simulink subsystem "EncondersHFz"  (R2023b)
settings: Solver=VariableStepAuto  StartTime=0.0  StopTime=10.0  RelTol=1e-3
libraries: arduinosensorlib x2, simulink x1
settings Model: Creator=Hajar  LastModifiedBy=Hajar

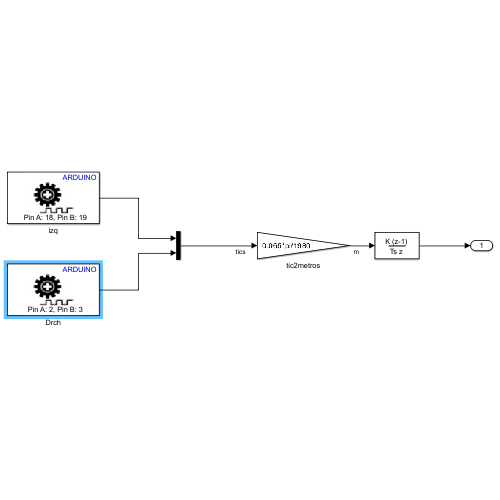
[thumbnail: Simulink's stored preview of the top-level diagram]
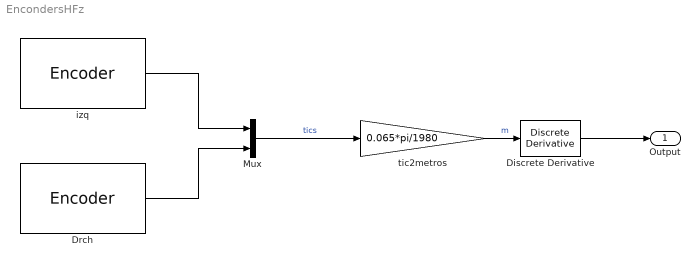
== system EncondersHFz ==
  Discrete Derivative : simulink/Discrete/Discrete Derivative  gainval=1.0  ICPrevScaledInput=0.0  OutMin=[]  OutMax=[]  OutDataType=fixdt(1, 16)  OutScaling=2^-10  DoSatur=off
  Drch : arduinosensorlib/Encoder  InputA=2  InputB=3  Mode=No reset  SampleTime=-1
  Mux : Mux  Inputs=2
  izq : arduinosensorlib/Encoder  InputA=18  InputB=19  Mode=No reset  SampleTime=-1
  tic2metros : Gain  Gain=0.065*pi/1980  OutDataTypeStr=double
  Output : Outport
  wires:
  izq/1 -> Mux/1
  Drch/1 -> Mux/2
  Mux/1 -> tic2metros/1  "tics"
  Discrete Derivative/1 -> Output/1
  tic2metros/1 -> Discrete Derivative/1  "m"
